simulink model "SS_model"  (R2020a)
settings: Solver=VariableStepAuto  StartTime=0.0  StopTime=100  RelTol=1e-3
values from neighbouring files (symbols this model uses):
  A = A_(2:end,2:end)    [state_space_equation.m]
  B = B_(2:end)    [state_space_equation.m]
  C = [1 0 0 ... (first row only)    [state_space_equation.m]
  K_ss = acker(A, B, des_pole)    [state_space_equation.m]
  x0 = [0 -ang 0]    [state_space_equation.m]
settings Model: Creator=Kian  LastModifiedBy=Kian

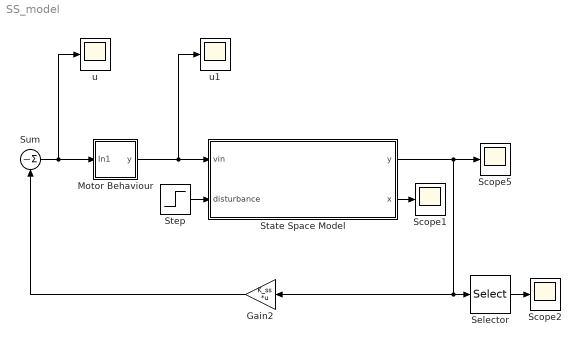
== system SS_model ==
  Gain2 : Gain  Gain=K_ss  Multiplication=Matrix(K*u)
  Motor Behaviour : Subsystem
  Scope1 : Scope
  Scope2 : Scope
  Scope5 : Scope
  Selector : Selector  InputPortWidth=3  IndexOptions=Index vector (dialog)  Indices=2  OutputSizes=1
  State Space Model : Subsystem
  Step : Step  After=0  SampleTime=0
  Sum : Sum  Inputs=|-
  u : Scope
  u1 : Scope
  wires:
  Gain2/1 -> Sum/1
  Step/1 -> State Space Model/2(disturbance)
  State Space Model/2(x) -> Scope1/1
  State Space Model/1(y) -> Scope5/1, Gain2/1, Selector/1
  Sum/1 -> Motor Behaviour/1(In1), u/1
  Motor Behaviour/1(y) -> u1/1, State Space Model/1(vin)
  Selector/1 -> Scope2/1

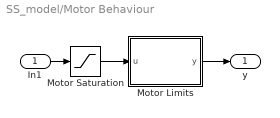
== system SS_model/Motor Behaviour ==
  In1 : Inport
  Motor Limits : MATLAB Function  TreatAsAtomicUnit=on
  Motor Saturation : Saturate  UpperLimit=10.5  LowerLimit=-10.5
  y : Outport
  wires:
  Motor Saturation/1 -> Motor Limits/1(u)
  In1/1 -> Motor Saturation/1
  Motor Limits/1(y) -> y/1

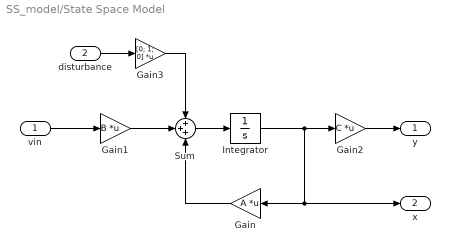
== system SS_model/State Space Model ==
  vin : Inport
  disturbance : Inport  Port=2
  Gain : Gain  Gain=A  Multiplication=Matrix(K*u)
  Gain1 : Gain  Gain=B  Multiplication=Matrix(K*u)
  Gain2 : Gain  Gain=C  Multiplication=Matrix(K*u)
  Gain3 : Gain  Gain=[0; 1; 0]  Multiplication=Matrix(K*u)
  Integrator : Integrator  InitialCondition=x0
  Sum : Sum  Inputs=+++
  y : Outport
  x : Outport  Port=2
  wires:
  Gain/1 -> Sum/3
  Sum/1 -> Integrator/1
  Gain1/1 -> Sum/2
  vin/1 -> Gain1/1
  Gain2/1 -> y/1
  Integrator/1 -> x/1, Gain/1, Gain2/1
  disturbance/1 -> Gain3/1
  Gain3/1 -> Sum/1

== matlab function SS_model/Motor Behaviour/Motor Limits ==
  data: u input; y output
function y = fcn(u)
deadzone = 3.5;

if sign(u) == 0
    y = 0;
elseif u*sign(u)<deadzone
    y = deadzone*sign(u);
else
    y = u;
end
